simulink model "conversion_mixing_matrix"  (R2019b)
settings: Solver=FixedStepAuto  StartTime=0.0  StopTime=10.0  RelTol=1e-3
undefined symbols (not defined in the file): g, m, max_T
settings Model: Creator=francois  LastModifiedBy=francois

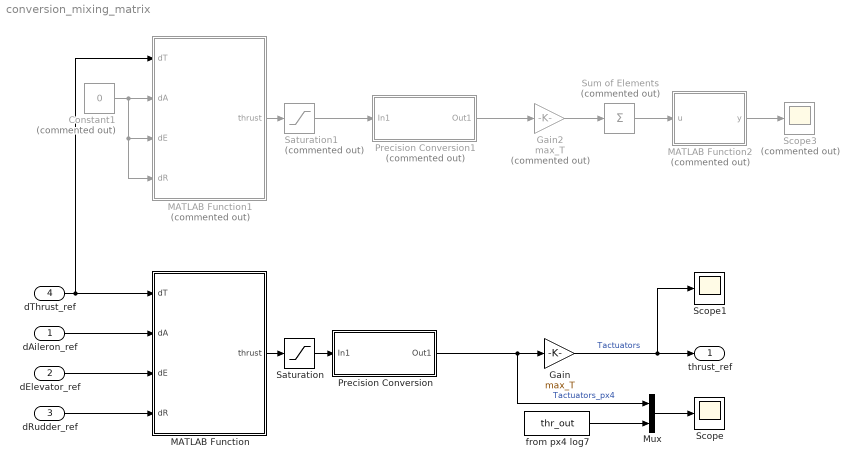
== system conversion_mixing_matrix ==
  dAileron_ref : Inport
  dElevator_ref : Inport  Port=2
  "dRudder_ref " : Inport  Port=3
  dThrust_ref : Inport  Port=4
  Constant1 : Constant  Commented=on  Value=0
  Gain : Gain  Gain=max_T
  Gain2 : Gain  Commented=on  Gain=max_T
  MATLAB Function : MATLAB Function  TreatAsAtomicUnit=on
  MATLAB Function1 : MATLAB Function  Commented=on  TreatAsAtomicUnit=on
  MATLAB Function2 : MATLAB Function  Commented=on  TreatAsAtomicUnit=on
  Mux : Mux  Inputs=2
  Precision Conversion : Subsystem
  Precision Conversion1 : Subsystem  Commented=on
  Saturation : Saturate  UpperLimit=1  LowerLimit=0
  Saturation1 : Saturate  Commented=on  UpperLimit=1  LowerLimit=0
  Scope : Scope
  Scope1 : Scope
  Scope3 : Scope  Commented=on
  Sum of Elements : Sum  Commented=on  Inputs=+
  from px4 log7 : FromWorkspace  VariableName=thr_out  SampleTime=0
  thrust_ref : Outport  VectorParamsAs1DForOutWhenUnconnected=off
  wires:
  Precision Conversion/1(Out1) -> Mux/1, Gain/1  "Tactuators_px4"
  dThrust_ref/1 -> MATLAB Function1/1(dT), MATLAB Function/1(dT)
  MATLAB Function/1(thrust) -> Saturation/1
  Precision Conversion1/1(Out1) -> Gain2/1
  Constant1/1 -> MATLAB Function1/4(dR), MATLAB Function1/3(dE), MATLAB Function1/2(dA)
  Gain2/1 -> Sum of Elements/1
  Gain/1 -> Scope1/1, thrust_ref/1  "Tactuators"
  Sum of Elements/1 -> MATLAB Function2/1(u)
  MATLAB Function2/1(y) -> Scope3/1
  from px4 log7/1 -> Mux/2
  Saturation1/1 -> Precision Conversion1/1(In1)
  Mux/1 -> Scope/1
  "dRudder_ref "/1 -> MATLAB Function/4(dR)
  Saturation/1 -> Precision Conversion/1(In1)
  dElevator_ref/1 -> MATLAB Function/3(dE)
  dAileron_ref/1 -> MATLAB Function/2(dA)
  MATLAB Function1/1(thrust) -> Saturation1/1

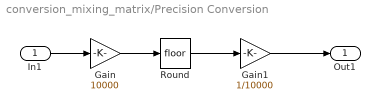
== system conversion_mixing_matrix/Precision Conversion ==
  In1 : Inport
  Gain : Gain  Gain=10000
  Gain1 : Gain  Gain=1/10000
  Round : Rounding
  Out1 : Outport  VectorParamsAs1DForOutWhenUnconnected=off
  wires:
  In1/1 -> Gain/1
  Gain/1 -> Round/1
  Round/1 -> Gain1/1
  Gain1/1 -> Out1/1

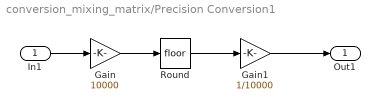
== system conversion_mixing_matrix/Precision Conversion1 ==
  In1 : Inport
  Gain : Gain  Gain=10000
  Gain1 : Gain  Gain=1/10000
  Round : Rounding
  Out1 : Outport  VectorParamsAs1DForOutWhenUnconnected=off
  wires:
  In1/1 -> Gain/1
  Gain/1 -> Round/1
  Round/1 -> Gain1/1
  Gain1/1 -> Out1/1

== matlab function conversion_mixing_matrix/MATLAB Function1 ==
  data: dT input; thrust output; dA input; dE input; dR input; mixin_mat parameter
function thrust = mixin_mat(dT, dA, dE, dR, mixin_mat)

    thrust = mixin_mat * [dT; dA; dE; dR];

end

== matlab function conversion_mixing_matrix/MATLAB Function ==
  data: dT input; thrust output; dA input; dE input; dR input; mixing_matrix parameter
function thrust = mixing_mat(dT, dA, dE, dR, mixing_matrix)

    thrust = mixing_matrix * [dT; dA; dE; dR];

end

== matlab function conversion_mixing_matrix/MATLAB Function2 ==
  data: u input; y output; m parameter; g parameter
function y = fcn(u, m, g)
    y = m/(1/((u/(m*g)) - 1) - 1);
end
